simulink model "iot_casestudy_1_2"  (R2023a)
settings: Solver=VariableStepAuto  StartTime=0.0  StopTime=3.0  RelTol=1e-3
undefined symbols (not defined in the file or in its folder): m, n
settings Model: PacingRate=0.089000  Creator=simon  LastModifiedBy=simon
settings DataIOCC: SignalLogging=off
settings OptimizationCC: AccelVerboseBuild=on

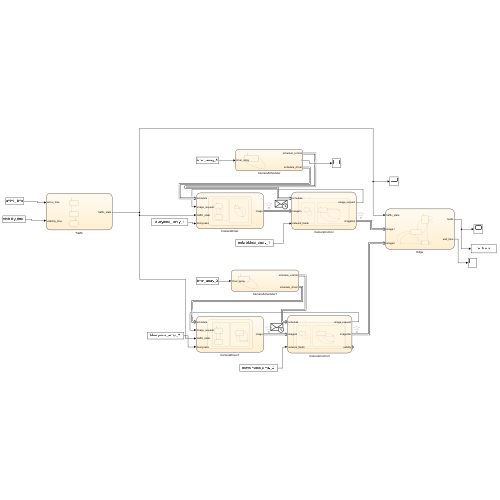
[thumbnail: Simulink's stored preview of the top-level diagram]
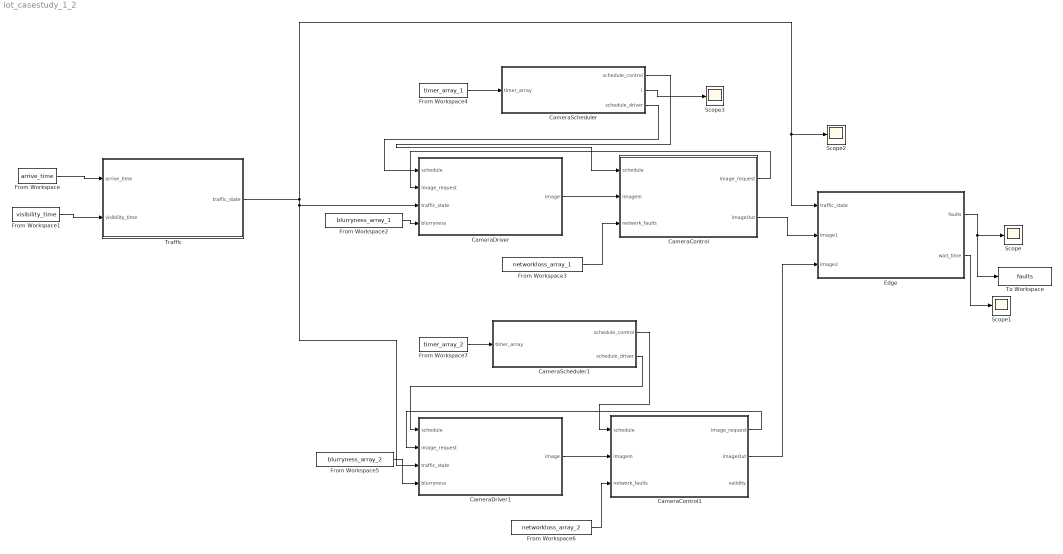
== system iot_casestudy_1_2 ==
  CameraControl : Stateflow chart  TreatAsAtomicUnit=on
      settings: PortSchema="{\"entries\":[{\"content\":{\"sides\":[{\"content\":{\"connectorIds\":[\"In3\",\"In1\",\"In2\"]},\"type\":\"ConnectorPlacement.EquallySpacedRectSide\",\"uuid\":\"ab620818-a51b-4a3c-9b00-600c4a6c30a0\"},{\"content\":{\"connectorIds\":[\"Out1\",\"Out2\"],\"side\":\"RIGHT\"},\"type\":\"ConnectorPlacement.EquallySpacedRectSide\",\"uuid\":\"fd7d4612-1aa1-44dc-acf4-0ffdcf3f06ab\"},{\"content\":{\"side\":\"TOP\"},\"type\":\"ConnectorPlacement.EquallySpacedRectSide\",\"uuid\":\"b173ad78-f658-4e97-9d6b-ed1d410de5f1\"}]},\"type\":\"ConnectorPlacement.EquallySpacedConnector\",\"uuid\":\"5700aeec-8725-4d1d-b13d-0f47828af58c\"}],\"packageUris\":[\"http://schema.mathworks.com/mf0/Connector/R2020b\"],\"version\":\"1.0\"}"
  CameraControl1 : Stateflow chart  TreatAsAtomicUnit=on
      settings: PortSchema="{\"entries\":[{\"content\":{\"sides\":[{\"content\":{\"connectorIds\":[\"In3\",\"In1\",\"In2\"]},\"type\":\"ConnectorPlacement.EquallySpacedRectSide\",\"uuid\":\"ab620818-a51b-4a3c-9b00-600c4a6c30a0\"},{\"content\":{\"connectorIds\":[\"Out1\",\"Out2\",\"Out3\"],\"side\":\"RIGHT\"},\"type\":\"ConnectorPlacement.EquallySpacedRectSide\",\"uuid\":\"fd7d4612-1aa1-44dc-acf4-0ffdcf3f06ab\"},{\"content\":{\"side\":\"TOP\"},\"type\":\"ConnectorPlacement.EquallySpacedRectSide\",\"uuid\":\"b173ad78-f658-4e97-9d6b-ed1d410de5f1\"}]},\"type\":\"ConnectorPlacement.EquallySpacedConnector\",\"uuid\":\"5700aeec-8725-4d1d-b13d-0f47828af58c\"}],\"packageUris\":[\"http://schema.mathworks.com/mf0/Connector/R2020b\"],\"version\":\"1.0\"}"
  CameraDriver : Stateflow chart  TreatAsAtomicUnit=on
      settings: PortSchema="{\"entries\":[{\"content\":{\"sides\":[{\"content\":{\"connectorIds\":[\"In4\",\"In1\",\"In2\",\"In3\"]},\"type\":\"ConnectorPlacement.EquallySpacedRectSide\",\"uuid\":\"49bdffc0-8e15-4462-b991-b36534669558\"},{\"content\":{\"connectorIds\":[\"Out1\"],\"side\":\"RIGHT\"},\"type\":\"ConnectorPlacement.EquallySpacedRectSide\",\"uuid\":\"379950e5-a8e3-41fb-8f45-c3d731cfbd8a\"},{\"content\":{\"side\":\"TOP\"},\"type\":\"ConnectorPlacement.EquallySpacedRectSide\",\"uuid\":\"38309075-1b62-4fbc-9171-ddac584f70df\"}]},\"type\":\"ConnectorPlacement.EquallySpacedConnector\",\"uuid\":\"335a78c7-f6bb-4aff-a350-269f860e2554\"}],\"packageUris\":[\"http://schema.mathworks.com/mf0/Connector/R2020b\"],\"version\":\"1.0\"}"
  CameraDriver1 : Stateflow chart  TreatAsAtomicUnit=on
      settings: PortSchema="{\"entries\":[{\"content\":{\"sides\":[{\"content\":{\"connectorIds\":[\"In4\",\"In1\",\"In2\",\"In3\"]},\"type\":\"ConnectorPlacement.EquallySpacedRectSide\",\"uuid\":\"49bdffc0-8e15-4462-b991-b36534669558\"},{\"content\":{\"connectorIds\":[\"Out1\"],\"side\":\"RIGHT\"},\"type\":\"ConnectorPlacement.EquallySpacedRectSide\",\"uuid\":\"379950e5-a8e3-41fb-8f45-c3d731cfbd8a\"},{\"content\":{\"side\":\"TOP\"},\"type\":\"ConnectorPlacement.EquallySpacedRectSide\",\"uuid\":\"38309075-1b62-4fbc-9171-ddac584f70df\"}]},\"type\":\"ConnectorPlacement.EquallySpacedConnector\",\"uuid\":\"335a78c7-f6bb-4aff-a350-269f860e2554\"}],\"packageUris\":[\"http://schema.mathworks.com/mf0/Connector/R2020b\"],\"version\":\"1.0\"}"
  CameraScheduler : Stateflow chart  TreatAsAtomicUnit=on
      settings: PortSchema="{\"entries\":[{\"content\":{\"sides\":[{\"content\":{\"connectorIds\":[\"In1\"]},\"type\":\"ConnectorPlacement.EquallySpacedRectSide\",\"uuid\":\"228150a7-62a2-46d0-a1ac-a8e868d835b5\"},{\"content\":{\"connectorIds\":[\"Out2\",\"Out3\",\"Out1\"],\"side\":\"RIGHT\"},\"type\":\"ConnectorPlacement.EquallySpacedRectSide\",\"uuid\":\"cb1c6840-c5bf-4913-92c2-1c054d368f87\"},{\"content\":{\"side\":\"TOP\"},\"type\":\"ConnectorPlacement.EquallySpacedRectSide\",\"uuid\":\"3633cd87-b3f9-48c9-80b7-73d7f17aa7ad\"}]},\"type\":\"ConnectorPlacement.EquallySpacedConnector\",\"uuid\":\"2553d532-cb7a-499b-b98c-b91f81677a07\"}],\"packageUris\":[\"http://schema.mathworks.com/mf0/Connector/R2020b\"],\"version\":\"1.0\"}"
  CameraScheduler1 : Stateflow chart  TreatAsAtomicUnit=on
      settings: PortSchema="{\"entries\":[{\"content\":{\"sides\":[{\"content\":{\"connectorIds\":[\"In1\"]},\"type\":\"ConnectorPlacement.EquallySpacedRectSide\",\"uuid\":\"335362b2-4c4f-40e6-baf0-d287f6971824\"},{\"content\":{\"connectorIds\":[\"Out2\",\"Out1\"],\"side\":\"RIGHT\"},\"type\":\"ConnectorPlacement.EquallySpacedRectSide\",\"uuid\":\"7ee54d08-aa3e-4d6f-8253-6f749626479a\"},{\"content\":{\"side\":\"TOP\"},\"type\":\"ConnectorPlacement.EquallySpacedRectSide\",\"uuid\":\"7bf47310-47f4-4483-b0d1-b8a087b66b77\"}]},\"type\":\"ConnectorPlacement.EquallySpacedConnector\",\"uuid\":\"fb61df21-9632-41f0-9cfa-ce5060944b6c\"}],\"packageUris\":[\"http://schema.mathworks.com/mf0/Connector/R2020b\"],\"version\":\"1.0\"}"
  Edge : Stateflow chart  TreatAsAtomicUnit=on
  From Workspace : FromWorkspace  VariableName=arrive_time  OutDataTypeStr=double  SampleTime=-1  Interpolate=off  ZeroCross=off  OutputAfterFinalValue=Holding final value
  From Workspace1 : FromWorkspace  VariableName=visibility_time  OutDataTypeStr=double  SampleTime=-1  Interpolate=off  ZeroCross=off  OutputAfterFinalValue=Holding final value
  From Workspace2 : FromWorkspace  VariableName=blurryness_array_1
  From Workspace3 : FromWorkspace  VariableName=networkloss_array_1
  From Workspace4 : FromWorkspace  VariableName=timer_array_1
  From Workspace5 : FromWorkspace  VariableName=blurryness_array_2
  From Workspace6 : FromWorkspace  VariableName=networkloss_array_2
  From Workspace7 : FromWorkspace  VariableName=timer_array_2
  Scope{,1..3} (4 alike) : Scope
  To Workspace : ToWorkspace  VariableName=faults  SaveFormat=Timeseries  SampleTime=-1
  Traffic : Stateflow chart  TreatAsAtomicUnit=on
  wires:
  From Workspace/1 -> Traffic/1(arrive_time)
  From Workspace1/1 -> Traffic/2(visibility_time)
  From Workspace2/1 -> CameraDriver/3(blurryness)
  CameraControl/1(image_request) -> CameraDriver/1(image_request)
  From Workspace3/1 -> CameraControl/2(network_faults)
  From Workspace4/1 -> CameraScheduler/1(timer_array)
  CameraDriver/1(image) -> CameraControl/1(imageIn)
  Edge/1(faults) -> Scope/1, To Workspace/1
  CameraControl1/2(imageOut) -> Edge/3(image2)
  CameraDriver1/1(image) -> CameraControl1/1(imageIn)
  From Workspace7/1 -> CameraScheduler1/1(timer_array)
  From Workspace6/1 -> CameraControl1/2(network_faults)
  CameraControl1/1(image_request) -> CameraDriver1/1(image_request)
  Traffic/1(traffic_state) -> Scope2/1, Edge/1(traffic_state), CameraDriver1/2(traffic_state), CameraDriver/2(traffic_state)
  From Workspace5/1 -> CameraDriver1/3(blurryness)
  CameraControl/2(imageOut) -> Edge/2(image1)
  CameraScheduler/1(schedule_driver) -> CameraDriver/4(schedule)
  CameraScheduler1/2(schedule_control) -> CameraControl1/3(schedule)
  CameraScheduler1/1(schedule_driver) -> CameraDriver1/4(schedule)
  CameraScheduler/2(schedule_control) -> CameraControl/3(schedule)
  Edge/2(wait_time) -> Scope1/1
  CameraScheduler/3(i) -> Scope3/1

== stateflow chart iot_casestudy_1_2/CameraScheduler ==
  settings: updateMethod=CONTINUOUS  executeAtInitialization=1
  state Main
    entry:
    dt=timer_array[i];
  state CascadeState
  (default) -> Main : {i=1;dt=0;}
  Main -> CascadeState : after(dt,msec){i=i+1;send(schedule_driver);}
  CascadeState -> Main : after(1,msec){send(schedule_control);}
  data: timer_array input; schedule_driver output double; schedule_control output double; dt local double; dt2 local double; i output double =0.0

== stateflow chart iot_casestudy_1_2/CameraControl1 ==
  settings: updateMethod=CONTINUOUS
  state Operation
    state RequestHangling [parallel]
      settings: executionOrder=1
      note: {image_request=1;}
      state Operation1
      (default) -> Operation1
      Operation1 -> Operation1 : schedule{image_request=1;}
    state ImageMessaging [parallel]
      settings: executionOrder=2
      state Operation2
        entry:
        validity=isvalid(imageIn);
      (default) -> Operation2 : {i=1;}
      (junction 29) -> Operation2 [order 1] : [i>0]
          | {receive(imageIn);i = i + 1;
          | imageOut.data=imageIn.data;
          | send(imageOut);}
      (junction 19) -> Operation2 [order 2] : {receive(imageIn);i = i + 1;}
      Operation2 -> (junction 19) : schedule
      (junction 29) -> Operation2 [order 2] : {i = i + 1;receive(imageIn);}
      (junction 19) -> (junction 29) [order 1] : [network_faults(i)==0]
  (default) -> Operation
  data: image_request output; imageIn input; i local; network_faults input; imageOut output; schedule input; validity output

== stateflow chart iot_casestudy_1_2/CameraDriver1 ==
  settings: updateMethod=CONTINUOUS
  state Operation
    state CarVisibility [parallel]
      settings: executionOrder=1
      state NoCar
        entry: car=0;
      state Car
        entry: car=1;
      (default) -> NoCar
      NoCar -> Car : [traffic_state==1]
      Car -> NoCar : [traffic_state==0]
    state DriverOperation [parallel]
      settings: executionOrder=2
      state Main
      (default) -> Main : {i=1;}
      Main -> (junction 22) : schedule
      (junction 22) -> Main [order 1] : [(car==1)&&(blurryness(i)==1)]
          | {image.data=1;send(image);i = i + 1;}
      (junction 22) -> Main [order 2] : {image.data=0;
          | send(image);i = i + 1;}
  data: image_request input; traffic_state input; blurryness input; image output; car local; i local; schedule input

== stateflow chart iot_casestudy_1_2/CameraScheduler1 ==
  settings: updateMethod=CONTINUOUS  executeAtInitialization=1
  state Main
    entry:
    dt=timer_array[i];
  state CascadeState
  (default) -> Main : {i=0;dt=0;}
  Main -> CascadeState : after(dt,msec){i=i+1;send(schedule_driver);}
  CascadeState -> Main : after(1,msec){send(schedule_control);}
  data: timer_array input; i local double; schedule_driver output double; schedule_control output double; dt local double

== stateflow chart iot_casestudy_1_2/CameraDriver ==
  settings: updateMethod=CONTINUOUS
  state Operation
    state CarVisibility [parallel]
      settings: executionOrder=1
      state NoCar
        entry: car=0;
      state Car
        entry: car=1;
      (default) -> NoCar
      NoCar -> Car : [traffic_state==1]
      Car -> NoCar : [traffic_state==0]
    state DriverOperation [parallel]
      settings: executionOrder=2
      state Main
      (default) -> Main : {i=1;}
      Main -> (junction 22) : schedule
      (junction 22) -> Main [order 2] : {image.data=0;
          | send(image);i = i + 1;}
      (junction 22) -> Main [order 1] : [(car==1)&&(blurryness(i)==1)]
          | {image.data=1;i = i + 1;send(image);}
  data: image_request input; traffic_state input; blurryness input; image output; car local; i local; schedule input

== stateflow chart iot_casestudy_1_2/CameraControl ==
  settings: updateMethod=CONTINUOUS
  state Operation
    state RequestHangling [parallel]
      settings: executionOrder=1
      state Operation1
      (default) -> Operation1 : {image_request=1;}
      Operation1 -> Operation1 : schedule{image_request=1;}
    state ImageMessaging [parallel]
      settings: executionOrder=2
      state Operation2
        entry:
        validity=isvalid(imageIn);
      (default) -> Operation2 : {i=1;}
      (junction 28) -> Operation2 [order 1] : [i>0]
          | {receive(imageIn);i = i + 1;
          | imageOut.data=imageIn.data
          | send(imageOut);}
      (junction 28) -> Operation2 [order 2] : {i = i + 1;receive(imageIn);}
      (junction 19) -> (junction 28) [order 1] : [network_faults(i)==0]
      (junction 19) -> Operation2 [order 2] : {receive(imageIn);i = i + 1;}
      Operation2 -> (junction 19) : schedule
  (default) -> Operation
  data: image_request output; imageIn input; i local; network_faults input; imageOut output; schedule input; validity local

== stateflow chart iot_casestudy_1_2/Traffic ==
  settings: updateMethod=CONTINUOUS
  state Nocar
    entry:
    traffic_state=0;
  state Car
    entry:
    traffic_state=1;
  state Nocar1
    entry:
    traffic_state=0;
  (default) -> Nocar
  Nocar -> Car : after(arrive_time,msec)
  Car -> Nocar1 : after(visibility_time,msec)
  data: arrive_time input; visibility_time input; traffic_state output

== stateflow chart iot_casestudy_1_2/Edge ==
  state Waiting
  state NotRecognized
    wait_time=elapsed(msec);
  state Recognized
  (default) -> Waiting : {faults=0;}
  Waiting -> Waiting [order 1] : image1{receive(image1);}
  Waiting -> NotRecognized [order 2] : [traffic_state==1]
  Waiting -> Waiting [order 3] : image2{receive(image2);}
  NotRecognized -> Waiting [order 1] : [traffic_state==0]
      | {faults=1;}
  Recognized -> Waiting [order 1] : [traffic_state==0]
  (junction 22) -> NotRecognized [order 2]
  NotRecognized -> (junction 22) [order 2] : image2
      | {receive(image2);}
  (junction 10) -> NotRecognized [order 2]
  NotRecognized -> (junction 10) [order 3] : image1{receive(image1);}
  (junction 10) -> Recognized [order 1] : [image1.data==1]
  Recognized -> Recognized [order 2] : image1{receive(image1);}
  Recognized -> Recognized [order 3] : image2{receive(image2);}
  (junction 22) -> Recognized [order 1] : [image2.data==1]
  data: traffic_state input; image1 input; faults output; image2 input; wait_time output
